simulink model "motor_controle_velocidade_simples"  (R2019b)
settings: Solver=VariableStepAuto  StartTime=0.0  StopTime=7  RelTol=1e-3
settings Model: Creator=fernandopassold  LastModifiedBy=fernandopassold

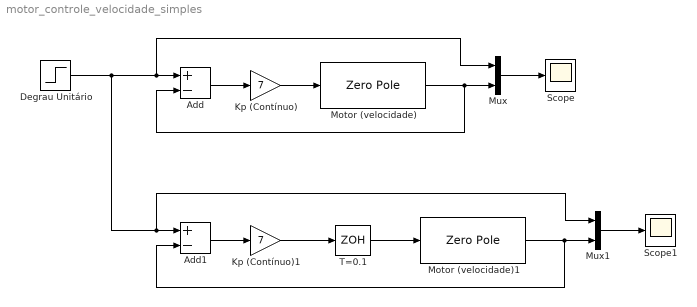
== system motor_controle_velocidade_simples ==
  Add : Sum  Inputs=+-
  Add1 : Sum  Inputs=+-
  Degrau Unitário : Step  SampleTime=0
  Kp (Contínuo) : Gain  Gain=7
  Kp (Contínuo)1 : Gain  Gain=7
  Motor (velocidade) : ZeroPole  Zeros=[]  Poles=[-2 -1/2]
  Motor (velocidade)1 : ZeroPole  Zeros=[]  Poles=[-2 -1/2]
  Mux : Mux  Inputs=2
  Mux1 : Mux  Inputs=2
  Scope : Scope
  Scope1 : Scope
  T=0.1 : ZeroOrderHold  SampleTime=0.1
  wires:
  Add/1 -> Kp (Contínuo)/1
  Kp (Contínuo)/1 -> Motor (velocidade)/1
  Motor (velocidade)/1 -> Add/2, Mux/2
  Mux/1 -> Scope/1
  Degrau Unitário/1 -> Mux1/1, Add1/1, Mux/1, Add/1
  Motor (velocidade)1/1 -> Add1/2, Mux1/2
  Add1/1 -> Kp (Contínuo)1/1
  Mux1/1 -> Scope1/1
  Kp (Contínuo)1/1 -> T=0.1/1
  T=0.1/1 -> Motor (velocidade)1/1
